simulink model "InternalADC20190225"  (R2018b)
settings: Solver=FixedStepDiscrete  StartTime=0.0  StopTime=Inf  RelTol=1e-3  EnableMultiTasking=on
undefined symbols (not defined in the file or in its folder): Down, GPTRIP1SEL, GPTRIP2SEL, TZ1, TZ2, Up
libraries: idelinklib_common x72, c2802xlib x32, c2837xDlib x32, simulink x16, c2000lib x1
(part 4 of 4)

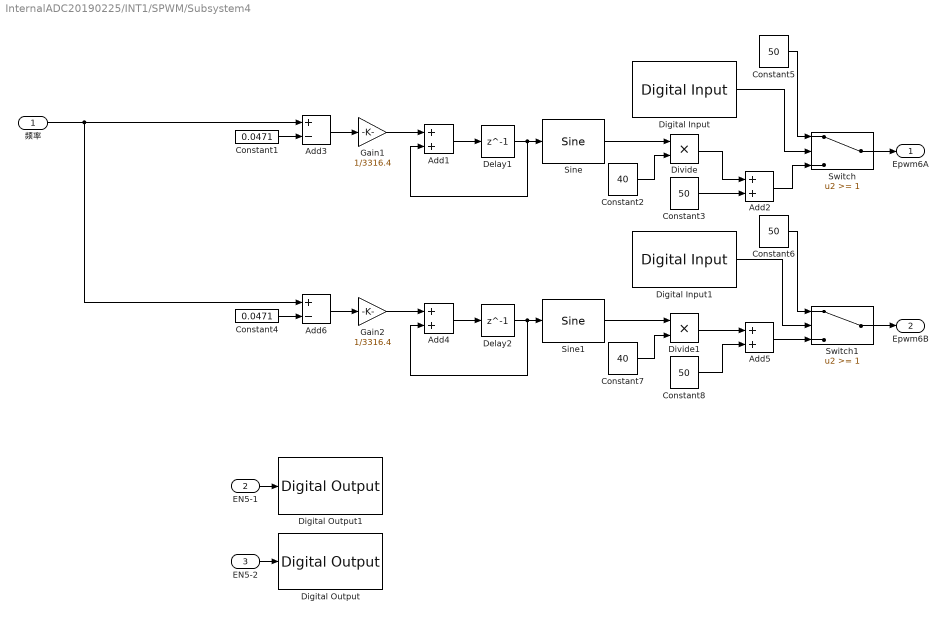
== system InternalADC20190225/INT1/SPWM/Subsystem4 ==
  频率 : Inport
  EN5-1 : Inport  Port=2
  EN5-2 : Inport  Port=3
  Add{1..2,4..5} (4 alike) : Sum
  Add3 : Sum  Inputs=+-
  Add6 : Sum  Inputs=+-
  Constant1 : Constant  Value=0.0471  VectorParams1D=off
  Constant2 : Constant  Value=40  VectorParams1D=off
  Constant{3,5..6,8} (4 alike) : Constant  Value=50  VectorParams1D=off
  Constant4 : Constant  Value=0.0471  VectorParams1D=off
  Constant7 : Constant  Value=40  VectorParams1D=off
  Delay1 : Delay  DelayLength=1
  Delay2 : Delay  DelayLength=1
  Digital Input : c2837xDlib/Digital Input  GPIO_Number=GPIO96~GPIO103  GPIO_Bit0=off  GPIO_Bit1=off  GPIO_Bit2=off  GPIO_Bit3=on  GPIO_Bit4=off  GPIO_Bit5=off  GPIO_Bit6=off  GPIO_Bit7=off  sampleTime=-1  dataType=auto  GPIO_Bit0_Qualification=Sync to SYSCLKOUT  GPIO_Bit1_Qualification=Sync to SYSCLKOUT  GPIO_Bit2_Qualification=Sync to SYSCLKOUT  GPIO_Bit3_Qualification=Sync to SYSCLKOUT  GPIO_Bit4_Qualification=Sync to SYSCLKOUT  GPIO_Bit5_Qualification=Sync to SYSCLKOUT  GPIO_Bit6_Qualification=Sync to SYSCLKOUT  GPIO_Bit7_Qualification=Sync to SYSCLKOUT  Qualification_Period=-1
      settings: SourceProductName=Embedded Coder Support Package for Texas Instruments C2000 Processors  SourceProductBaseCode=TIC2000
  Digital Input1 : c2837xDlib/Digital Input  GPIO_Number=GPIO96~GPIO103  GPIO_Bit0=off  GPIO_Bit1=off  GPIO_Bit2=off  GPIO_Bit3=on  GPIO_Bit4=off  GPIO_Bit5=off  GPIO_Bit6=off  GPIO_Bit7=off  sampleTime=-1  dataType=auto  GPIO_Bit0_Qualification=Sync to SYSCLKOUT  GPIO_Bit1_Qualification=Sync to SYSCLKOUT  GPIO_Bit2_Qualification=Sync to SYSCLKOUT  GPIO_Bit3_Qualification=Sync to SYSCLKOUT  GPIO_Bit4_Qualification=Sync to SYSCLKOUT  GPIO_Bit5_Qualification=Sync to SYSCLKOUT  GPIO_Bit6_Qualification=Sync to SYSCLKOUT  GPIO_Bit7_Qualification=Sync to SYSCLKOUT  Qualification_Period=-1
      settings: SourceProductName=Embedded Coder Support Package for Texas Instruments C2000 Processors  SourceProductBaseCode=TIC2000
  Digital Output : c2837xDlib/Digital Output  GPIO_Number=GPIO88~GPIO95  GPIO_Bit0=off  GPIO_BIT0_Toggle=off  GPIO_Bit1=off  GPIO_BIT1_Toggle=off  GPIO_Bit2=off  GPIO_BIT2_Toggle=off  GPIO_Bit3=on  GPIO_BIT3_Toggle=off  GPIO_Bit4=off  GPIO_BIT4_Toggle=off  GPIO_Bit5=off  GPIO_BIT5_Toggle=off  GPIO_Bit6=off  GPIO_BIT6_Toggle=off  GPIO_Bit7=off  GPIO_BIT7_Toggle=off
      settings: SourceProductName=Embedded Coder Support Package for Texas Instruments C2000 Processors  SourceProductBaseCode=TIC2000
  Digital Output1 : c2837xDlib/Digital Output  GPIO_Number=GPIO88~GPIO95  GPIO_Bit0=off  GPIO_BIT0_Toggle=off  GPIO_Bit1=off  GPIO_BIT1_Toggle=off  GPIO_Bit2=off  GPIO_BIT2_Toggle=off  GPIO_Bit3=off  GPIO_BIT3_Toggle=off  GPIO_Bit4=on  GPIO_BIT4_Toggle=off  GPIO_Bit5=off  GPIO_BIT5_Toggle=off  GPIO_Bit6=off  GPIO_BIT6_Toggle=off  GPIO_Bit7=off  GPIO_BIT7_Toggle=off
      settings: SourceProductName=Embedded Coder Support Package for Texas Instruments C2000 Processors  SourceProductBaseCode=TIC2000
  Divide : Product  Inputs=**
  Divide1 : Product  Inputs=**
  Gain1 : Gain  Gain=1/3316.4
  Gain2 : Gain  Gain=1/3316.4
  Sine : simulink/Lookup Tables/Sine  Formula=sin(2*pi*u)  NumDataPoints=(2^8)+1  OutputWordLength=16  InternalRulePriority=Speed
      settings: SourceProductName=Simulink
  Sine1 : simulink/Lookup Tables/Sine  Formula=sin(2*pi*u)  NumDataPoints=(2^8)+1  OutputWordLength=16  InternalRulePriority=Speed
      settings: SourceProductName=Simulink
  Switch : Switch  Threshold=1
  Switch1 : Switch  Threshold=1
  Epwm6A : Outport
  Epwm6B : Outport  Port=2
  wires:
  EN5-2/1 -> Digital Output/1
  EN5-1/1 -> Digital Output1/1
  频率/1 -> Add3/1, Add6/1
  Digital Input/1 -> Switch/2
  Switch/1 -> Epwm6A/1
  Sine/1 -> Divide/1
  Delay2/1 -> Add4/2, Sine1/1
  Constant1/1 -> Add3/2
  Add4/1 -> Delay2/1
  Add3/1 -> Gain1/1
  Constant2/1 -> Divide/2
  Constant8/1 -> Add5/2
  Constant7/1 -> Divide1/2
  Gain2/1 -> Add4/1
  Sine1/1 -> Divide1/1
  Add6/1 -> Gain2/1
  Constant4/1 -> Add6/2
  Delay1/1 -> Sine/1, Add1/2
  Add1/1 -> Delay1/1
  Digital Input1/1 -> Switch1/2
  Switch1/1 -> Epwm6B/1
  Add5/1 -> Switch1/3
  Gain1/1 -> Add1/1
  Add2/1 -> Switch/3
  Constant6/1 -> Switch1/1
  Divide/1 -> Add2/1
  Divide1/1 -> Add5/1
  Constant3/1 -> Add2/2
  Constant5/1 -> Switch/1

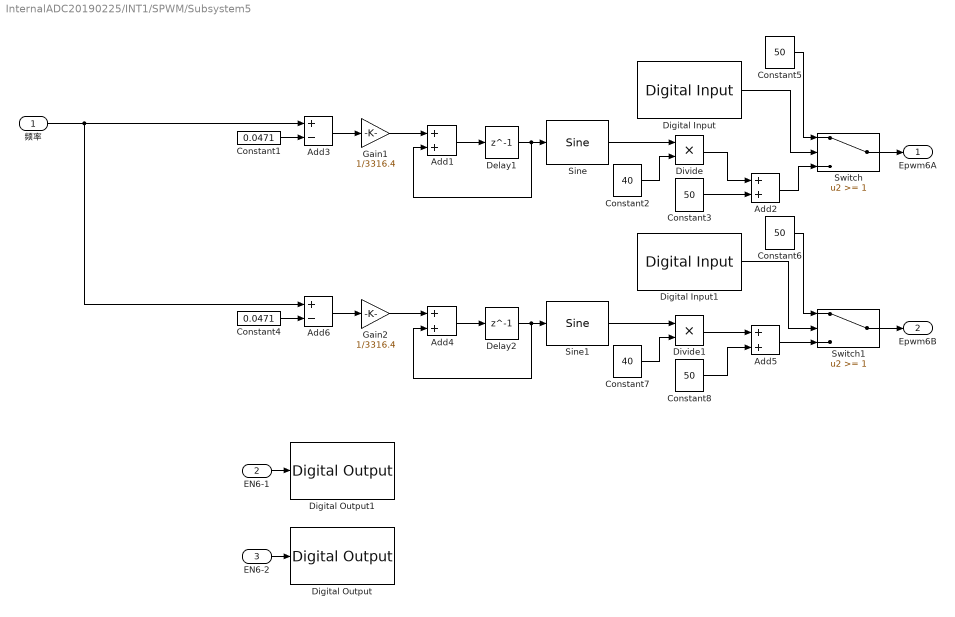
== system InternalADC20190225/INT1/SPWM/Subsystem5 ==
  频率 : Inport
  EN6-1 : Inport  Port=2
  EN6-2 : Inport  Port=3
  Add{1..2,4..5} (4 alike) : Sum
  Add3 : Sum  Inputs=+-
  Add6 : Sum  Inputs=+-
  Constant1 : Constant  Value=0.0471  VectorParams1D=off
  Constant2 : Constant  Value=40  VectorParams1D=off
  Constant{3,5..6,8} (4 alike) : Constant  Value=50  VectorParams1D=off
  Constant4 : Constant  Value=0.0471  VectorParams1D=off
  Constant7 : Constant  Value=40  VectorParams1D=off
  Delay1 : Delay  DelayLength=1
  Delay2 : Delay  DelayLength=1
  Digital Input : c2837xDlib/Digital Input  GPIO_Number=GPIO96~GPIO103  GPIO_Bit0=off  GPIO_Bit1=off  GPIO_Bit2=off  GPIO_Bit3=on  GPIO_Bit4=off  GPIO_Bit5=off  GPIO_Bit6=off  GPIO_Bit7=off  sampleTime=-1  dataType=auto  GPIO_Bit0_Qualification=Sync to SYSCLKOUT  GPIO_Bit1_Qualification=Sync to SYSCLKOUT  GPIO_Bit2_Qualification=Sync to SYSCLKOUT  GPIO_Bit3_Qualification=Sync to SYSCLKOUT  GPIO_Bit4_Qualification=Sync to SYSCLKOUT  GPIO_Bit5_Qualification=Sync to SYSCLKOUT  GPIO_Bit6_Qualification=Sync to SYSCLKOUT  GPIO_Bit7_Qualification=Sync to SYSCLKOUT  Qualification_Period=-1
      settings: SourceProductName=Embedded Coder Support Package for Texas Instruments C2000 Processors  SourceProductBaseCode=TIC2000
  Digital Input1 : c2837xDlib/Digital Input  GPIO_Number=GPIO96~GPIO103  GPIO_Bit0=off  GPIO_Bit1=off  GPIO_Bit2=off  GPIO_Bit3=on  GPIO_Bit4=off  GPIO_Bit5=off  GPIO_Bit6=off  GPIO_Bit7=off  sampleTime=-1  dataType=auto  GPIO_Bit0_Qualification=Sync to SYSCLKOUT  GPIO_Bit1_Qualification=Sync to SYSCLKOUT  GPIO_Bit2_Qualification=Sync to SYSCLKOUT  GPIO_Bit3_Qualification=Sync to SYSCLKOUT  GPIO_Bit4_Qualification=Sync to SYSCLKOUT  GPIO_Bit5_Qualification=Sync to SYSCLKOUT  GPIO_Bit6_Qualification=Sync to SYSCLKOUT  GPIO_Bit7_Qualification=Sync to SYSCLKOUT  Qualification_Period=-1
      settings: SourceProductName=Embedded Coder Support Package for Texas Instruments C2000 Processors  SourceProductBaseCode=TIC2000
  Digital Output : c2837xDlib/Digital Output  GPIO_Number=GPIO88~GPIO95  GPIO_Bit0=off  GPIO_BIT0_Toggle=off  GPIO_Bit1=on  GPIO_BIT1_Toggle=off  GPIO_Bit2=off  GPIO_BIT2_Toggle=off  GPIO_Bit3=off  GPIO_BIT3_Toggle=off  GPIO_Bit4=off  GPIO_BIT4_Toggle=off  GPIO_Bit5=off  GPIO_BIT5_Toggle=off  GPIO_Bit6=off  GPIO_BIT6_Toggle=off  GPIO_Bit7=off  GPIO_BIT7_Toggle=off
      settings: SourceProductName=Embedded Coder Support Package for Texas Instruments C2000 Processors  SourceProductBaseCode=TIC2000
  Digital Output1 : c2837xDlib/Digital Output  GPIO_Number=GPIO88~GPIO95  GPIO_Bit0=off  GPIO_BIT0_Toggle=off  GPIO_Bit1=off  GPIO_BIT1_Toggle=off  GPIO_Bit2=on  GPIO_BIT2_Toggle=off  GPIO_Bit3=off  GPIO_BIT3_Toggle=off  GPIO_Bit4=off  GPIO_BIT4_Toggle=off  GPIO_Bit5=off  GPIO_BIT5_Toggle=off  GPIO_Bit6=off  GPIO_BIT6_Toggle=off  GPIO_Bit7=off  GPIO_BIT7_Toggle=off
      settings: SourceProductName=Embedded Coder Support Package for Texas Instruments C2000 Processors  SourceProductBaseCode=TIC2000
  Divide : Product  Inputs=**
  Divide1 : Product  Inputs=**
  Gain1 : Gain  Gain=1/3316.4
  Gain2 : Gain  Gain=1/3316.4
  Sine : simulink/Lookup Tables/Sine  Formula=sin(2*pi*u)  NumDataPoints=(2^8)+1  OutputWordLength=16  InternalRulePriority=Speed
      settings: SourceProductName=Simulink
  Sine1 : simulink/Lookup Tables/Sine  Formula=sin(2*pi*u)  NumDataPoints=(2^8)+1  OutputWordLength=16  InternalRulePriority=Speed
      settings: SourceProductName=Simulink
  Switch : Switch  Threshold=1
  Switch1 : Switch  Threshold=1
  Epwm6A : Outport
  Epwm6B : Outport  Port=2
  wires:
  EN6-1/1 -> Digital Output1/1
  EN6-2/1 -> Digital Output/1
  频率/1 -> Add3/1, Add6/1
  Digital Input/1 -> Switch/2
  Switch/1 -> Epwm6A/1
  Sine/1 -> Divide/1
  Delay2/1 -> Add4/2, Sine1/1
  Constant1/1 -> Add3/2
  Add4/1 -> Delay2/1
  Add3/1 -> Gain1/1
  Constant2/1 -> Divide/2
  Constant8/1 -> Add5/2
  Constant7/1 -> Divide1/2
  Gain2/1 -> Add4/1
  Sine1/1 -> Divide1/1
  Add6/1 -> Gain2/1
  Constant4/1 -> Add6/2
  Delay1/1 -> Sine/1, Add1/2
  Add1/1 -> Delay1/1
  Digital Input1/1 -> Switch1/2
  Switch1/1 -> Epwm6B/1
  Add5/1 -> Switch1/3
  Gain1/1 -> Add1/1
  Add2/1 -> Switch/3
  Constant6/1 -> Switch1/1
  Divide/1 -> Add2/1
  Divide1/1 -> Add5/1
  Constant3/1 -> Add2/2
  Constant5/1 -> Switch/1

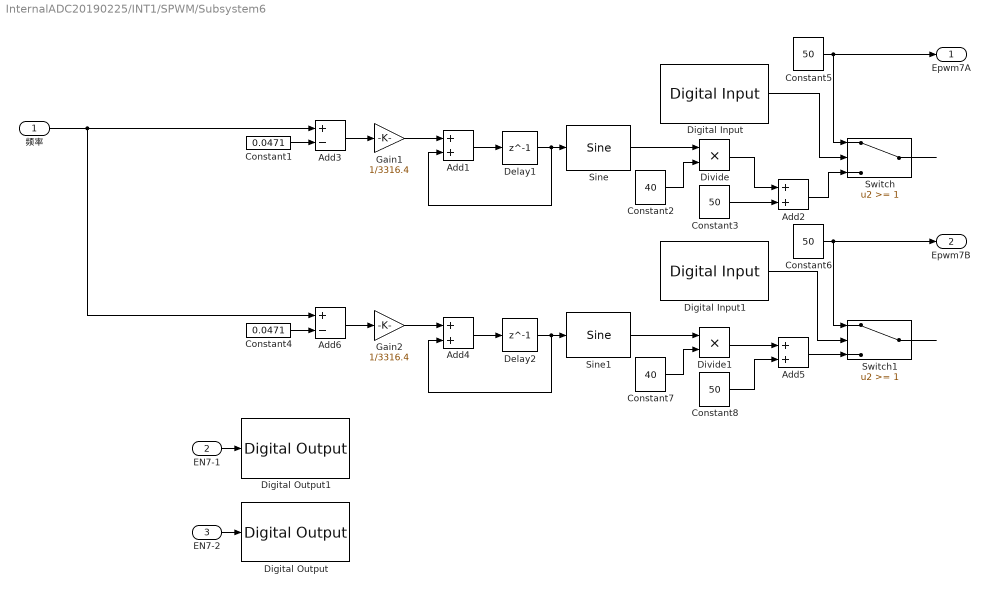
== system InternalADC20190225/INT1/SPWM/Subsystem6 ==
  频率 : Inport
  EN7-1 : Inport  Port=2
  EN7-2 : Inport  Port=3
  Add{1..2,4..5} (4 alike) : Sum
  Add3 : Sum  Inputs=+-
  Add6 : Sum  Inputs=+-
  Constant1 : Constant  Value=0.0471  VectorParams1D=off
  Constant2 : Constant  Value=40  VectorParams1D=off
  Constant{3,5..6,8} (4 alike) : Constant  Value=50  VectorParams1D=off
  Constant4 : Constant  Value=0.0471  VectorParams1D=off
  Constant7 : Constant  Value=40  VectorParams1D=off
  Delay1 : Delay  DelayLength=1
  Delay2 : Delay  DelayLength=1
  Digital Input : c2837xDlib/Digital Input  GPIO_Number=GPIO96~GPIO103  GPIO_Bit0=off  GPIO_Bit1=off  GPIO_Bit2=off  GPIO_Bit3=on  GPIO_Bit4=off  GPIO_Bit5=off  GPIO_Bit6=off  GPIO_Bit7=off  sampleTime=-1  dataType=auto  GPIO_Bit0_Qualification=Sync to SYSCLKOUT  GPIO_Bit1_Qualification=Sync to SYSCLKOUT  GPIO_Bit2_Qualification=Sync to SYSCLKOUT  GPIO_Bit3_Qualification=Sync to SYSCLKOUT  GPIO_Bit4_Qualification=Sync to SYSCLKOUT  GPIO_Bit5_Qualification=Sync to SYSCLKOUT  GPIO_Bit6_Qualification=Sync to SYSCLKOUT  GPIO_Bit7_Qualification=Sync to SYSCLKOUT  Qualification_Period=-1
      settings: SourceProductName=Embedded Coder Support Package for Texas Instruments C2000 Processors  SourceProductBaseCode=TIC2000
  Digital Input1 : c2837xDlib/Digital Input  GPIO_Number=GPIO96~GPIO103  GPIO_Bit0=off  GPIO_Bit1=off  GPIO_Bit2=off  GPIO_Bit3=on  GPIO_Bit4=off  GPIO_Bit5=off  GPIO_Bit6=off  GPIO_Bit7=off  sampleTime=-1  dataType=auto  GPIO_Bit0_Qualification=Sync to SYSCLKOUT  GPIO_Bit1_Qualification=Sync to SYSCLKOUT  GPIO_Bit2_Qualification=Sync to SYSCLKOUT  GPIO_Bit3_Qualification=Sync to SYSCLKOUT  GPIO_Bit4_Qualification=Sync to SYSCLKOUT  GPIO_Bit5_Qualification=Sync to SYSCLKOUT  GPIO_Bit6_Qualification=Sync to SYSCLKOUT  GPIO_Bit7_Qualification=Sync to SYSCLKOUT  Qualification_Period=-1
      settings: SourceProductName=Embedded Coder Support Package for Texas Instruments C2000 Processors  SourceProductBaseCode=TIC2000
  Digital Output : c2837xDlib/Digital Output  GPIO_Number=GPIO80~GPIO87  GPIO_Bit0=off  GPIO_BIT0_Toggle=off  GPIO_Bit1=off  GPIO_BIT1_Toggle=off  GPIO_Bit2=off  GPIO_BIT2_Toggle=off  GPIO_Bit3=off  GPIO_BIT3_Toggle=off  GPIO_Bit4=off  GPIO_BIT4_Toggle=off  GPIO_Bit5=off  GPIO_BIT5_Toggle=off  GPIO_Bit6=off  GPIO_BIT6_Toggle=off  GPIO_Bit7=on  GPIO_BIT7_Toggle=off
      settings: SourceProductName=Embedded Coder Support Package for Texas Instruments C2000 Processors  SourceProductBaseCode=TIC2000
  Digital Output1 : c2837xDlib/Digital Output  GPIO_Number=GPIO88~GPIO95  GPIO_Bit0=on  GPIO_BIT0_Toggle=off  GPIO_Bit1=off  GPIO_BIT1_Toggle=off  GPIO_Bit2=off  GPIO_BIT2_Toggle=off  GPIO_Bit3=off  GPIO_BIT3_Toggle=off  GPIO_Bit4=off  GPIO_BIT4_Toggle=off  GPIO_Bit5=off  GPIO_BIT5_Toggle=off  GPIO_Bit6=off  GPIO_BIT6_Toggle=off  GPIO_Bit7=off  GPIO_BIT7_Toggle=off
      settings: SourceProductName=Embedded Coder Support Package for Texas Instruments C2000 Processors  SourceProductBaseCode=TIC2000
  Divide : Product  Inputs=**
  Divide1 : Product  Inputs=**
  Gain1 : Gain  Gain=1/3316.4
  Gain2 : Gain  Gain=1/3316.4
  Sine : simulink/Lookup Tables/Sine  Formula=sin(2*pi*u)  NumDataPoints=(2^8)+1  OutputWordLength=16  InternalRulePriority=Speed
      settings: SourceProductName=Simulink
  Sine1 : simulink/Lookup Tables/Sine  Formula=sin(2*pi*u)  NumDataPoints=(2^8)+1  OutputWordLength=16  InternalRulePriority=Speed
      settings: SourceProductName=Simulink
  Switch : Switch  Threshold=1
  Switch1 : Switch  Threshold=1
  Epwm7A : Outport
  Epwm7B : Outport  Port=2
  wires:
  EN7-1/1 -> Digital Output1/1
  EN7-2/1 -> Digital Output/1
  频率/1 -> Add3/1, Add6/1
  Digital Input/1 -> Switch/2
  Switch/1 -> ?
  Sine/1 -> Divide/1
  Delay2/1 -> Add4/2, Sine1/1
  Constant1/1 -> Add3/2
  Add4/1 -> Delay2/1
  Add3/1 -> Gain1/1
  Constant2/1 -> Divide/2
  Constant8/1 -> Add5/2
  Constant7/1 -> Divide1/2
  Gain2/1 -> Add4/1
  Sine1/1 -> Divide1/1
  Add6/1 -> Gain2/1
  Constant4/1 -> Add6/2
  Delay1/1 -> Sine/1, Add1/2
  Add1/1 -> Delay1/1
  Digital Input1/1 -> Switch1/2
  Switch1/1 -> ?
  Add5/1 -> Switch1/3
  Gain1/1 -> Add1/1
  Add2/1 -> Switch/3
  Constant6/1 -> Epwm7B/1, Switch1/1
  Divide/1 -> Add2/1
  Divide1/1 -> Add5/1
  Constant3/1 -> Add2/2
  Constant5/1 -> Switch/1, Epwm7A/1

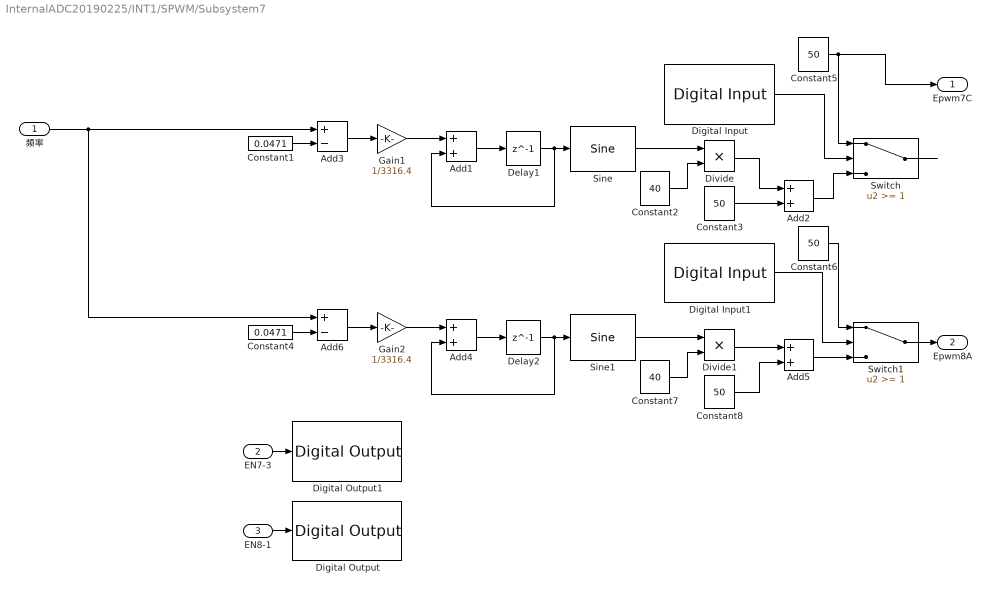
== system InternalADC20190225/INT1/SPWM/Subsystem7 ==
  频率 : Inport
  EN7-3 : Inport  Port=2
  EN8-1 : Inport  Port=3
  Add{1..2,4..5} (4 alike) : Sum
  Add3 : Sum  Inputs=+-
  Add6 : Sum  Inputs=+-
  Constant1 : Constant  Value=0.0471  VectorParams1D=off
  Constant2 : Constant  Value=40  VectorParams1D=off
  Constant{3,5..6,8} (4 alike) : Constant  Value=50  VectorParams1D=off
  Constant4 : Constant  Value=0.0471  VectorParams1D=off
  Constant7 : Constant  Value=40  VectorParams1D=off
  Delay1 : Delay  DelayLength=1
  Delay2 : Delay  DelayLength=1
  Digital Input : c2837xDlib/Digital Input  GPIO_Number=GPIO96~GPIO103  GPIO_Bit0=off  GPIO_Bit1=off  GPIO_Bit2=off  GPIO_Bit3=on  GPIO_Bit4=off  GPIO_Bit5=off  GPIO_Bit6=off  GPIO_Bit7=off  sampleTime=-1  dataType=auto  GPIO_Bit0_Qualification=Sync to SYSCLKOUT  GPIO_Bit1_Qualification=Sync to SYSCLKOUT  GPIO_Bit2_Qualification=Sync to SYSCLKOUT  GPIO_Bit3_Qualification=Sync to SYSCLKOUT  GPIO_Bit4_Qualification=Sync to SYSCLKOUT  GPIO_Bit5_Qualification=Sync to SYSCLKOUT  GPIO_Bit6_Qualification=Sync to SYSCLKOUT  GPIO_Bit7_Qualification=Sync to SYSCLKOUT  Qualification_Period=-1
      settings: SourceProductName=Embedded Coder Support Package for Texas Instruments C2000 Processors  SourceProductBaseCode=TIC2000
  Digital Input1 : c2837xDlib/Digital Input  GPIO_Number=GPIO96~GPIO103  GPIO_Bit0=off  GPIO_Bit1=off  GPIO_Bit2=off  GPIO_Bit3=on  GPIO_Bit4=off  GPIO_Bit5=off  GPIO_Bit6=off  GPIO_Bit7=off  sampleTime=-1  dataType=auto  GPIO_Bit0_Qualification=Sync to SYSCLKOUT  GPIO_Bit1_Qualification=Sync to SYSCLKOUT  GPIO_Bit2_Qualification=Sync to SYSCLKOUT  GPIO_Bit3_Qualification=Sync to SYSCLKOUT  GPIO_Bit4_Qualification=Sync to SYSCLKOUT  GPIO_Bit5_Qualification=Sync to SYSCLKOUT  GPIO_Bit6_Qualification=Sync to SYSCLKOUT  GPIO_Bit7_Qualification=Sync to SYSCLKOUT  Qualification_Period=-1
      settings: SourceProductName=Embedded Coder Support Package for Texas Instruments C2000 Processors  SourceProductBaseCode=TIC2000
  Digital Output : c2837xDlib/Digital Output  GPIO_Number=GPIO48~GPIO55  GPIO_Bit0=off  GPIO_BIT0_Toggle=off  GPIO_Bit1=off  GPIO_BIT1_Toggle=off  GPIO_Bit2=off  GPIO_BIT2_Toggle=off  GPIO_Bit3=off  GPIO_BIT3_Toggle=off  GPIO_Bit4=on  GPIO_BIT4_Toggle=off  GPIO_Bit5=off  GPIO_BIT5_Toggle=off  GPIO_Bit6=off  GPIO_BIT6_Toggle=off  GPIO_Bit7=off  GPIO_BIT7_Toggle=off
      settings: SourceProductName=Embedded Coder Support Package for Texas Instruments C2000 Processors  SourceProductBaseCode=TIC2000
  Digital Output1 : c2837xDlib/Digital Output  GPIO_Number=GPIO80~GPIO87  GPIO_Bit0=off  GPIO_BIT0_Toggle=off  GPIO_Bit1=off  GPIO_BIT1_Toggle=off  GPIO_Bit2=off  GPIO_BIT2_Toggle=off  GPIO_Bit3=off  GPIO_BIT3_Toggle=off  GPIO_Bit4=off  GPIO_BIT4_Toggle=off  GPIO_Bit5=off  GPIO_BIT5_Toggle=off  GPIO_Bit6=on  GPIO_BIT6_Toggle=off  GPIO_Bit7=off  GPIO_BIT7_Toggle=off
      settings: SourceProductName=Embedded Coder Support Package for Texas Instruments C2000 Processors  SourceProductBaseCode=TIC2000
  Divide : Product  Inputs=**
  Divide1 : Product  Inputs=**
  Gain1 : Gain  Gain=1/3316.4
  Gain2 : Gain  Gain=1/3316.4
  Sine : simulink/Lookup Tables/Sine  Formula=sin(2*pi*u)  NumDataPoints=(2^8)+1  OutputWordLength=16  InternalRulePriority=Speed
      settings: SourceProductName=Simulink
  Sine1 : simulink/Lookup Tables/Sine  Formula=sin(2*pi*u)  NumDataPoints=(2^8)+1  OutputWordLength=16  InternalRulePriority=Speed
      settings: SourceProductName=Simulink
  Switch : Switch  Threshold=1
  Switch1 : Switch  Threshold=1
  Epwm7C : Outport
  Epwm8A : Outport  Port=2
  wires:
  EN8-1/1 -> Digital Output/1
  EN7-3/1 -> Digital Output1/1
  频率/1 -> Add3/1, Add6/1
  Digital Input/1 -> Switch/2
  Switch/1 -> ?
  Sine/1 -> Divide/1
  Delay2/1 -> Add4/2, Sine1/1
  Constant1/1 -> Add3/2
  Add4/1 -> Delay2/1
  Add3/1 -> Gain1/1
  Constant2/1 -> Divide/2
  Constant8/1 -> Add5/2
  Constant7/1 -> Divide1/2
  Gain2/1 -> Add4/1
  Sine1/1 -> Divide1/1
  Add6/1 -> Gain2/1
  Constant4/1 -> Add6/2
  Delay1/1 -> Sine/1, Add1/2
  Add1/1 -> Delay1/1
  Digital Input1/1 -> Switch1/2
  Switch1/1 -> Epwm8A/1
  Add5/1 -> Switch1/3
  Gain1/1 -> Add1/1
  Add2/1 -> Switch/3
  Constant6/1 -> Switch1/1
  Divide/1 -> Add2/1
  Divide1/1 -> Add5/1
  Constant3/1 -> Add2/2
  Constant5/1 -> Epwm7C/1, Switch/1

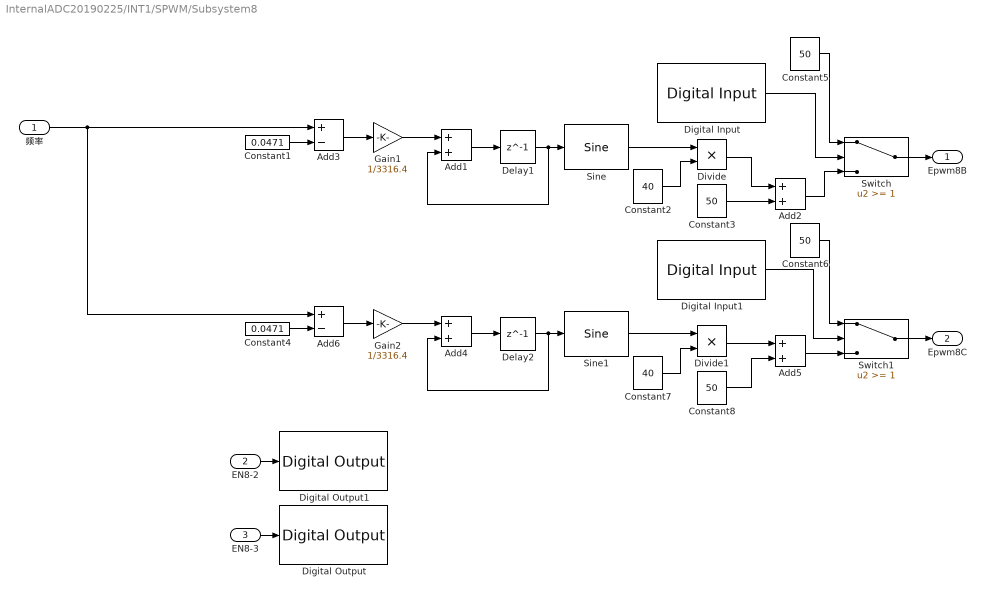
== system InternalADC20190225/INT1/SPWM/Subsystem8 ==
  频率 : Inport
  EN8-2 : Inport  Port=2
  EN8-3 : Inport  Port=3
  Add{1..2,4..5} (4 alike) : Sum
  Add3 : Sum  Inputs=+-
  Add6 : Sum  Inputs=+-
  Constant1 : Constant  Value=0.0471  VectorParams1D=off
  Constant2 : Constant  Value=40  VectorParams1D=off
  Constant{3,5..6,8} (4 alike) : Constant  Value=50  VectorParams1D=off
  Constant4 : Constant  Value=0.0471  VectorParams1D=off
  Constant7 : Constant  Value=40  VectorParams1D=off
  Delay1 : Delay  DelayLength=1
  Delay2 : Delay  DelayLength=1
  Digital Input : c2837xDlib/Digital Input  GPIO_Number=GPIO96~GPIO103  GPIO_Bit0=off  GPIO_Bit1=off  GPIO_Bit2=off  GPIO_Bit3=on  GPIO_Bit4=off  GPIO_Bit5=off  GPIO_Bit6=off  GPIO_Bit7=off  sampleTime=-1  dataType=auto  GPIO_Bit0_Qualification=Sync to SYSCLKOUT  GPIO_Bit1_Qualification=Sync to SYSCLKOUT  GPIO_Bit2_Qualification=Sync to SYSCLKOUT  GPIO_Bit3_Qualification=Sync to SYSCLKOUT  GPIO_Bit4_Qualification=Sync to SYSCLKOUT  GPIO_Bit5_Qualification=Sync to SYSCLKOUT  GPIO_Bit6_Qualification=Sync to SYSCLKOUT  GPIO_Bit7_Qualification=Sync to SYSCLKOUT  Qualification_Period=-1
      settings: SourceProductName=Embedded Coder Support Package for Texas Instruments C2000 Processors  SourceProductBaseCode=TIC2000
  Digital Input1 : c2837xDlib/Digital Input  GPIO_Number=GPIO96~GPIO103  GPIO_Bit0=off  GPIO_Bit1=off  GPIO_Bit2=off  GPIO_Bit3=on  GPIO_Bit4=off  GPIO_Bit5=off  GPIO_Bit6=off  GPIO_Bit7=off  sampleTime=-1  dataType=auto  GPIO_Bit0_Qualification=Sync to SYSCLKOUT  GPIO_Bit1_Qualification=Sync to SYSCLKOUT  GPIO_Bit2_Qualification=Sync to SYSCLKOUT  GPIO_Bit3_Qualification=Sync to SYSCLKOUT  GPIO_Bit4_Qualification=Sync to SYSCLKOUT  GPIO_Bit5_Qualification=Sync to SYSCLKOUT  GPIO_Bit6_Qualification=Sync to SYSCLKOUT  GPIO_Bit7_Qualification=Sync to SYSCLKOUT  Qualification_Period=-1
      settings: SourceProductName=Embedded Coder Support Package for Texas Instruments C2000 Processors  SourceProductBaseCode=TIC2000
  Digital Output : c2837xDlib/Digital Output  GPIO_Number=GPIO48~GPIO55  GPIO_Bit0=off  GPIO_BIT0_Toggle=off  GPIO_Bit1=off  GPIO_BIT1_Toggle=off  GPIO_Bit2=on  GPIO_BIT2_Toggle=off  GPIO_Bit3=off  GPIO_BIT3_Toggle=off  GPIO_Bit4=off  GPIO_BIT4_Toggle=off  GPIO_Bit5=off  GPIO_BIT5_Toggle=off  GPIO_Bit6=off  GPIO_BIT6_Toggle=off  GPIO_Bit7=off  GPIO_BIT7_Toggle=off
      settings: SourceProductName=Embedded Coder Support Package for Texas Instruments C2000 Processors  SourceProductBaseCode=TIC2000
  Digital Output1 : c2837xDlib/Digital Output  GPIO_Number=GPIO48~GPIO55  GPIO_Bit0=off  GPIO_BIT0_Toggle=off  GPIO_Bit1=off  GPIO_BIT1_Toggle=off  GPIO_Bit2=off  GPIO_BIT2_Toggle=off  GPIO_Bit3=on  GPIO_BIT3_Toggle=off  GPIO_Bit4=off  GPIO_BIT4_Toggle=off  GPIO_Bit5=off  GPIO_BIT5_Toggle=off  GPIO_Bit6=off  GPIO_BIT6_Toggle=off  GPIO_Bit7=off  GPIO_BIT7_Toggle=off
      settings: SourceProductName=Embedded Coder Support Package for Texas Instruments C2000 Processors  SourceProductBaseCode=TIC2000
  Divide : Product  Inputs=**
  Divide1 : Product  Inputs=**
  Gain1 : Gain  Gain=1/3316.4
  Gain2 : Gain  Gain=1/3316.4
  Sine : simulink/Lookup Tables/Sine  Formula=sin(2*pi*u)  NumDataPoints=(2^8)+1  OutputWordLength=16  InternalRulePriority=Speed
      settings: SourceProductName=Simulink
  Sine1 : simulink/Lookup Tables/Sine  Formula=sin(2*pi*u)  NumDataPoints=(2^8)+1  OutputWordLength=16  InternalRulePriority=Speed
      settings: SourceProductName=Simulink
  Switch : Switch  Threshold=1
  Switch1 : Switch  Threshold=1
  Epwm8B : Outport
  Epwm8C : Outport  Port=2
  wires:
  EN8-2/1 -> Digital Output1/1
  EN8-3/1 -> Digital Output/1
  频率/1 -> Add3/1, Add6/1
  Digital Input/1 -> Switch/2
  Switch/1 -> Epwm8B/1
  Sine/1 -> Divide/1
  Delay2/1 -> Add4/2, Sine1/1
  Constant1/1 -> Add3/2
  Add4/1 -> Delay2/1
  Add3/1 -> Gain1/1
  Constant2/1 -> Divide/2
  Constant8/1 -> Add5/2
  Constant7/1 -> Divide1/2
  Gain2/1 -> Add4/1
  Sine1/1 -> Divide1/1
  Add6/1 -> Gain2/1
  Constant4/1 -> Add6/2
  Delay1/1 -> Sine/1, Add1/2
  Add1/1 -> Delay1/1
  Digital Input1/1 -> Switch1/2
  Switch1/1 -> Epwm8C/1
  Add5/1 -> Switch1/3
  Gain1/1 -> Add1/1
  Add2/1 -> Switch/3
  Constant6/1 -> Switch1/1
  Divide/1 -> Add2/1
  Divide1/1 -> Add5/1
  Constant3/1 -> Add2/2
  Constant5/1 -> Switch/1
